simulink model "M1_P2_C"  (R2023a)
settings: Solver=VariableStepAuto  StartTime=0.0  StopTime=1  RelTol=1e-3
undefined symbols (not defined in the file): f_eff, J_eff, Kb, Ktn, L, R
settings Model: Creator=azzam  LastModifiedBy=azzam

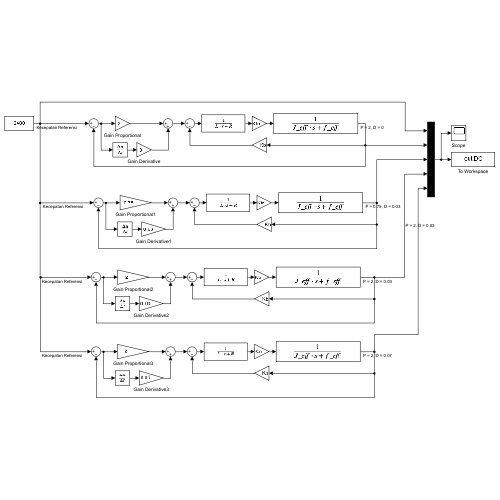
[thumbnail: Simulink's stored preview of the top-level diagram]
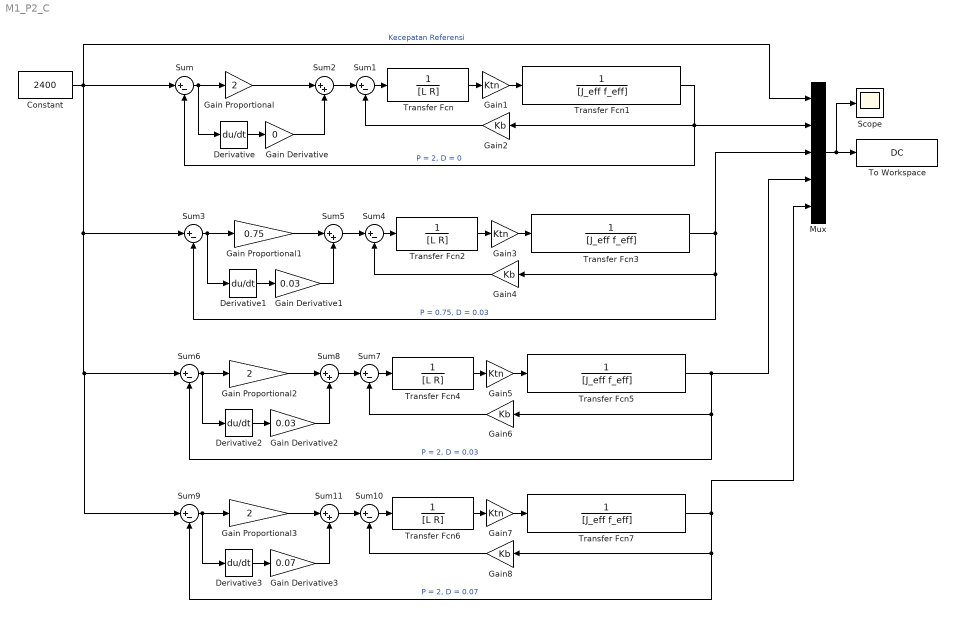
== system M1_P2_C ==
  Constant : Constant  Value=2400
  Derivative{,1..3} (4 alike) : Derivative
  Gain Derivative : Gain  Gain=0
  Gain Derivative1 : Gain  Gain=0.03
  Gain Derivative2 : Gain  Gain=0.03
  Gain Derivative3 : Gain  Gain=0.07
  Gain Proportional : Gain  Gain=2
  Gain Proportional1 : Gain  Gain=0.75
  Gain Proportional2 : Gain  Gain=2
  Gain Proportional3 : Gain  Gain=2
  Gain{1,3,5,7} (4 alike) : Gain  Gain=Ktn
  Gain{2,4,6,8} (4 alike) : Gain  Gain=Kb
  Mux : Mux  Inputs=5
  Scope : Scope
  Sum{,1,3..4,6..7,9..10} (8 alike) : Sum  Inputs=|+-
  Sum{2,5,8,11} (4 alike) : Sum  Inputs=|++
  To Workspace : ToWorkspace  VariableName=DC  SaveFormat=Timeseries  SampleTime=-1
  Transfer Fcn{,2,4,6} (4 alike) : TransferFcn  Denominator=[L R]
  Transfer Fcn{1,3,5,7} (4 alike) : TransferFcn  Denominator=[J_eff f_eff]
  wires:
  Sum2/1 -> Sum1/1
  Derivative/1 -> Gain Derivative/1
  Gain Derivative/1 -> Sum2/2
  Sum/1 -> Derivative/1, Gain Proportional/1
  Gain2/1 -> Sum1/2
  Transfer Fcn1/1 -> Mux/2, Gain2/1, Sum/2  "P = 2, D = 0"
  Transfer Fcn/1 -> Gain1/1
  Sum1/1 -> Transfer Fcn/1
  Gain Proportional/1 -> Sum2/1
  Gain1/1 -> Transfer Fcn1/1
  Mux/1 -> To Workspace/1, Scope/1
  Gain3/1 -> Transfer Fcn3/1
  Sum4/1 -> Transfer Fcn2/1
  Gain Proportional1/1 -> Sum5/1
  Derivative1/1 -> Gain Derivative1/1
  Transfer Fcn3/1 -> Gain4/1, Sum3/2, Mux/3  "P = 0.75, D = 0.03"
  Gain4/1 -> Sum4/2
  Gain Derivative1/1 -> Sum5/2
  Sum5/1 -> Sum4/1
  Transfer Fcn2/1 -> Gain3/1
  Sum3/1 -> Derivative1/1, Gain Proportional1/1
  Gain5/1 -> Transfer Fcn5/1
  Transfer Fcn5/1 -> Mux/4, Gain6/1, Sum6/2  "P = 2, D = 0.03"
  Derivative2/1 -> Gain Derivative2/1
  Gain Proportional2/1 -> Sum8/1
  Gain Derivative2/1 -> Sum8/2
  Gain6/1 -> Sum7/2
  Transfer Fcn4/1 -> Gain5/1
  Sum8/1 -> Sum7/1
  Sum6/1 -> Derivative2/1, Gain Proportional2/1
  Sum7/1 -> Transfer Fcn4/1
  Constant/1 -> Sum/1, Mux/1, Sum3/1, Sum6/1, Sum9/1  "Kecepatan Referensi"
  Gain7/1 -> Transfer Fcn7/1
  Transfer Fcn7/1 -> Mux/5, Gain8/1, Sum9/2  "P = 2, D = 0.07"
  Derivative3/1 -> Gain Derivative3/1
  Gain Proportional3/1 -> Sum11/1
  Gain Derivative3/1 -> Sum11/2
  Gain8/1 -> Sum10/2
  Transfer Fcn6/1 -> Gain7/1
  Sum11/1 -> Sum10/1
  Sum9/1 -> Derivative3/1, Gain Proportional3/1
  Sum10/1 -> Transfer Fcn6/1
